simulink model "model_16_09_22"  (R2021a)
settings: Solver=FixedStepAuto  StartTime=0.0  StopTime=1370  FixedStep=0.01  RelTol=1e-3
values from neighbouring files (symbols this model uses):
  coord_0_ecef = [x_0_ecef, y_0_ecef, z_0_ecef]    [new_path_local_frame4_05_2022.m]
  dampPitchConst = 5    [Configuration_13_09_22FINESTRELLE.m]
  dampRollConst = 5    [Configuration_13_09_22FINESTRELLE.m]
  ECC = 0.0818191908426    [new_path_local_frame4_05_2022.m]
  FsGong = 8192    [matlabSounds.mat]
  FsHandel = 8192    [matlabSounds.mat]
  gainPitchTorque = -1000    [Configuration_13_09_22FINESTRELLE.m]
  gainRollTorque = -1000    [Configuration_13_09_22FINESTRELLE.m]
  indirect = 1    [Configuration_13_09_22FINESTRELLE.m]
  R_E = 6378137    [new_path_local_frame4_05_2022.m]
  RotationMatrix_NWU2ECEF = [-cos(lon0)*sin(lat0),  sin(lon0), cos(lon0)*cos(lat0) ... (first row only)    [new_path_local_frame4_05_2022.m]
  springPitchConst = 35    [Configuration_13_09_22FINESTRELLE.m]
  springRollConst = 35    [Configuration_13_09_22FINESTRELLE.m]
  timesPitch = 0.6    [Configuration_13_09_22FINESTRELLE.m]
  timesRoll = 0.6    [Configuration_13_09_22FINESTRELLE.m]
  yGong = [-0.00269844839217 -0.00449741398696 -0.00742073307848 -0.011018664268 -0.0128176298628 -0.0173150438498 -0.0222621992354 -0.0222621992354 -0.020013492242 -0.00921969867326 0.00449741398696 0.0101191814707 ... (42028 elements, 42028x1)]    [matlabSounds.mat]
  yHandel = [0 -0.00615680615681 -0.0750360750361 -0.0311688311688 0.00615680615681 0.0380952380952 0.0188552188552 -0.025012025012 -0.0311688311688 -0.0750360750361 -0.12582972583 -0.1443001443 ... (73113 elements, 73113x1)]    [matlabSounds.mat]
undefined symbols (not defined in the file or in its folder): DiscIntNeverNeededParam, f
libraries: cstblocks x7, simulink x6, instrumentlib x5
(part 2 of 2)

== matlab function model_16_09_22/Controllers/BuildMessage ==
  data: springRoll output; commandRollDiretto input; commandPitchDiretto input; frictionRoll output; dampRoll output; torqueRoll output; springPitch output; frictionPitch output; dampPitch output; torquePitch output; springYaw output; frictionYaw output; dampYaw output; torqueYaw output; springRollConst parameter; dampRollConst parameter; dampPitchConst parameter; springPitchConst parameter
function [springRoll, frictionRoll, dampRoll, torqueRoll,...
          springPitch, frictionPitch, dampPitch, torquePitch,...
          springYaw, frictionYaw, dampYaw, torqueYaw] = fcn(commandRollDiretto,commandPitchDiretto, springRollConst,...
                                                            dampRollConst,dampPitchConst, springPitchConst)
    
    springRoll = springRollConst;
    frictionRoll = 0; 
    dampRoll= dampRollConst; 
    torqueRoll = commandRollDiretto;
    
    springPitch = springPitchConst;
    frictionPitch = 0; 
    dampPitch = dampPitchConst; 
    torquePitch = commandPitchDiretto;
    
    springYaw = 0; 
    frictionYaw = 0; 
    dampYaw = 0; 
    torqueYaw = 0;

== matlab function model_16_09_22/ComputeError/ToWorkspace3/MATLAB Function ==
  data: intersectionPoint input; intersectionPointX output; intersectionPointY output; intersectionPointhZ output
function [intersectionPointX, intersectionPointY, intersectionPointhZ] = split(intersectionPoint)
          intersectionPointX = intersectionPoint(1);
          intersectionPointY = intersectionPoint(2);
          intersectionPointhZ = intersectionPoint(3);

== matlab function model_16_09_22/ComputeError/ToWorkspace2/MATLAB Function1 ==
  data: coordclock input; coordclockX output; coordclockY output; coordclockZ output
function [coordclockX, coordclockY, coordclockZ] = split(coordclock)
          coordclockX = coordclock(1);
          coordclockY = coordclock(2);
          coordclockZ = coordclock(3);

== matlab function model_16_09_22/ComputeError/ToWorkspace1/MATLAB Function2 ==
  data: posAircraft input; posAircraftX output; posAircraftY output; posAircraftZ output
function [posAircraftX, posAircraftY, posAircraftZ] = split(posAircraft)
          posAircraftX = posAircraft(1);
          posAircraftY = posAircraft(2);
          posAircraftZ = posAircraft(3);

== matlab function model_16_09_22/Controllers/MATLAB Function ==
  data: springRoll input; DataSend output; frictionRoll input; dampRoll input; torqueRoll input; springPitch input; frictionPitch input; dampPitch input; torquePitch input; springYaw input; frictionYaw input; dampYaw input; torqueYaw input
function DataSend  = fcn(springRoll, frictionRoll, dampRoll, torqueRoll, springPitch, frictionPitch, dampPitch, torquePitch, springYaw, frictionYaw, dampYaw, torqueYaw)

DataSend = [springRoll, frictionRoll, dampRoll, torqueRoll, springPitch, frictionPitch, dampPitch, torquePitch, springYaw, frictionYaw, dampYaw, torqueYaw];

== matlab function model_16_09_22/Controllers/Pitch1 ==
  data: h input; distPitch output
function distPitch = fcn(h)
    %PITCH   
    deadZoneZ = 0;  %[m]
    
    y = h ;
    
    if ((abs(h) > deadZoneZ) && (h > 0))
        errorheight = abs(abs(y) - deadZoneZ);
    elseif ((abs(h) > deadZoneZ) && (h < 0))
        errorheight = - abs(abs(y) - deadZoneZ); %y<0
    else
        errorheight = 0;
    end
    
    distPitch = errorheight;

== matlab function model_16_09_22/MagnitudeReceive/logStickDeflection/MATLAB Function1 ==
  data: stickDeflection input; stickDeflectionX output; stickDeflectionY output; stickDeflectionZ output
function [stickDeflectionX, stickDeflectionY, stickDeflectionZ] = split(stickDeflection)
          stickDeflectionX = stickDeflection(1);
          stickDeflectionY = stickDeflection(2);
          stickDeflectionZ = stickDeflection(3);

== matlab function model_16_09_22/MagnitudeReceive/logMotorTorque/MATLAB Function1 ==
  data: motorTorqueVector input; motorTorqueX output; motorTorqueY output
function [motorTorqueX, motorTorqueY] = split(motorTorqueVector)
          motorTorqueX = motorTorqueVector(1);
          motorTorqueY = motorTorqueVector(2);

== matlab function model_16_09_22/MATLAB Function ==
  data: yGong parameter; FsGong parameter; start input; yHandel parameter; FsHandel parameter
function audio(yGong, FsGong, start, yHandel, FsHandel)
         coder.extrinsic('sound');
         %DA METTERE NELLO SCRIPT load matlabSounds.mat
         if start == 1  
            sound(yGong, FsGong);
         elseif start == 2
           sound(yHandel, FsHandel);
         end
         
         
         %play(p, [1 (get(p, 'SampleRate') * 3)]);

== matlab function model_16_09_22/timeAnalysis/MATLAB Function1 ==
  data: WINDOWStimeSec output
   function WINDOWStimeSec = sysClock()
       coder.extrinsic('clock');

       H  =  0;
       MN = 0;
       S  =  0;
       dateTime = clock;
       H  = dateTime(4);
       MN = dateTime(5);
       S  = dateTime(6);
       
       % secondi dall'inizio dell'ora corrente
       WINDOWStimeSec = S + MN*60;
       
   end

== matlab function model_16_09_22/timeAnalysis/deBiaser ==
  data: u input; y output
function y = deBias(u)
persistent initVal

if isempty(initVal)
    initVal = u;
end


y = u - initVal;

== matlab function model_16_09_22/timeAnalysis/deBiaser1 ==
  data: u input; y output
function y = deBias(u)
persistent initVal

if isempty(initVal)
    initVal = u;
end


y = u - initVal;

== matlab function model_16_09_22/timeAnalysis/deBiaser2 ==
  data: u input; y output
function y = deBias(u)
persistent initVal

if isempty(initVal)
    initVal = u;
end


y = u - initVal;

== matlab function model_16_09_22/timeAnalysis/deBiaser3 ==
  data: u input; y output
function y = deBias(u)
persistent initVal

if isempty(initVal)
    initVal = u;
end


y = u - initVal;

== matlab function model_16_09_22/timeAnalysis/deBiaser4 ==
  data: u input; y output
function y = deBias(u)
persistent initVal

if isempty(initVal)
    initVal = u;
end


y = u - initVal;

== matlab function model_16_09_22/MATLAB Function1 ==
  data: start input; FsGong parameter; yGong parameter; yHandel parameter; FsHandel parameter
function audio(start, FsGong, yGong, yHandel, FsHandel)
         coder.extrinsic('sound');
         %DA METTERE NELLO SCRIPT load matlabSounds.mat
         if start == 1  
            sound(yGong, FsGong);
         elseif start == 1365
           sound(yHandel, FsHandel);
         end
end

== matlab function model_16_09_22/CoordinatesConversions/MATLAB Function ==
  data: lat input; coord_ecef output; lon input; alt input; ECC parameter; R_E parameter
function coord_ecef = geo2ecef(lat, lon, alt, ECC, R_E)
    %THIS BLOCK IS JUST TO UNDERSTAND IF AEROFLY ECEF SYSTEM IS ORIENTED IN
    %THE SAME WAY AS I WOULD DO IT


    %we already have lat lon in radians
    %coord_geo = [lat, lon, alt];

%     normal radius
    N = R_E / sqrt(1 - (ECC * sin(lat))^2);

%     coordinate transformation
    x_ecef = (N + alt) * cos(lat) * cos(lon);
    y_ecef = (N + alt) * cos(lat) * sin(lon);
    z_ecef = (N * (1 - ECC^2) + alt) * sin(lat);

    coord_ecef = [x_ecef, y_ecef, z_ecef];
end

== matlab function model_16_09_22/split message ==
  data: u input; flight_time output; lat output; lon output; height output; roll output; pitch output; yaw output; coord_ecef_aerofly output; altitude output; controls_roll_input output; controls_pitch_input output; controls_yaw_input output; aircraft_aileron output; aircraft_elevator output; aircraft_velocityX output; aircraft_velocityY output; aircraft_velocityZ output; UDPcounter output
function [flight_time, lat, lon, height, roll, pitch, yaw, ...
          coord_ecef_aerofly, altitude,controls_roll_input, controls_pitch_input, controls_yaw_input,...
          aircraft_aileron, aircraft_elevator, aircraft_velocityX, aircraft_velocityY, aircraft_velocityZ, UDPcounter] = split(u)
 
 
%// send binary data to matlab TO COUNT IN MATLAB ADD 1
% 	gAircraftData2MatlabBuffer[0] = lfFlightTimeS;
% 
% 	gAircraftData2MatlabBuffer[1] = aircraft_position.x;
% 	gAircraftData2MatlabBuffer[2] = aircraft_position.y;
% 	gAircraftData2MatlabBuffer[3] = aircraft_position.z;
% 
% 	gAircraftData2MatlabBuffer[4] = aircraft_latitude;
% 	gAircraftData2MatlabBuffer[5] = aircraft_longitude;
% 
% 	gAircraftData2MatlabBuffer[6] = aircraft_height;
% 
% 	gAircraftData2MatlabBuffer[7] = aircraft_altitude;
% 
% 	gAircraftData2MatlabBuffer[8] = aircraft_bank;
% 	gAircraftData2MatlabBuffer[9] = aircraft_pitch;
% 	gAircraftData2MatlabBuffer[10] = aircraft_heading;
% 	gAircraftData2MatlabBuffer[11] = controls_roll_input;
% 	gAircraftData2MatlabBuffer[12] = controls_pitch_input;
% 	gAircraftData2MatlabBuffer[13] = controls_yaw_input;
% 	//gAircraftData2MatlabBuffer[14] = controls_roll_input_offset;
% 	//gAircraftData2MatlabBuffer[15] = controls_pitch_input_offset;
% 	gAircraftData2MatlabBuffer[14] = aircraft_aileron;
% 	gAircraftData2MatlabBuffer[15] = aircraft_elevator;
% 	gAircraftData2MatlabBuffer[16] = aircraft_velocity.x;
% 	gAircraftData2MatlabBuffer[17] = aircraft_velocity.y;
% 	gAircraftData2MatlabBuffer[18] = aircraft_velocity.z;
% 	
% 
% 	// ...
% 	gAircraftData2MatlabBuffer[19] = nUdpCounter;


    flight_time = u(1);
    x_pos = u(2);
    y_pos = u(3);
    z_pos = - u(4);
    coord_ecef_aerofly = [x_pos, y_pos, - z_pos];
    
    lat = u(5);
    lon = u(6);
    height = u(7);
    
    altitude = u(8);
    
    roll = rad2deg(u(9));
    pitch = - rad2deg(u(10));
    %pay attention the conversion is made just here and not in the logfile
    %this way the angle will be referred to the north and counted clockwise
    %for now we don't use it, but pay attention to the local frame and the
    %reference systems of the other angles if using them together for the
    %feedback
    yaw = 360 - rad2deg(u(11)) + 90;
    
    controls_roll_input = u(12);
    controls_pitch_input = u(13);
    controls_yaw_input = u(14);
        
    aircraft_aileron = u(15);
    aircraft_elevator = u(16);
    
    aircraft_velocityX = u(17);
    aircraft_velocityY = u(18);
    aircraft_velocityZ = u(19);
    
    UDPcounter = u(20);
    
    
end

== matlab function model_16_09_22/ComputeError/ToWorkspace4/MATLAB Function1 ==
  data: aircraft2path input; aircraft2pathX output; aircraft2pathY output; aircraft2pathZ output
function [aircraft2pathX, aircraft2pathY, aircraft2pathZ] = split(aircraft2path)
          aircraft2pathX = aircraft2path(1);
          aircraft2pathY = aircraft2path(2);
          aircraft2pathZ = aircraft2path(3);

== matlab function model_16_09_22/ComputeError/ComputeValidIndex ==
  data: startIndex output; stopIndex output; min_valid_index output; min_valid_theta output; min_valid_coord_path output; min_valid_tangent output; eps_Deg output; min_valid_aircraft2path output; norm_min_valid_aircraft2path output; g_Coordinates data_store_memory; plane_coord_nwu input; R parameter

function [startIndex, stopIndex, min_valid_index, ...
          min_valid_theta, min_valid_coord_path, min_valid_tangent, eps_Deg, ...
          min_valid_aircraft2path, norm_min_valid_aircraft2path] = fcn(plane_coord_nwu, R)

global g_Coordinates
persistent p_epsDeg; if isempty(p_epsDeg) p_epsDeg = 120.0; end
persistent p_prev_min_index ; if isempty(p_prev_min_index) p_prev_min_index = 1; end
persistent p_act_min_index ; if isempty(p_act_min_index) p_act_min_index = 1; end
persistent p_start; if isempty(p_start) p_start = true; end
persistent p_tangent_min; if isempty(p_tangent_min) p_tangent_min = [0, 0, 0]; end
persistent p_coord_path_min; if isempty(p_coord_path_min) p_coord_path_min = [0, 0, 0]; end
persistent p_min_valid_aircraft2path; if isempty(p_min_valid_aircraft2path) p_min_valid_aircraft2path = [0, 0, 0]; end

nSteps = g_Coordinates.Steps;

%init some variables
n90DegCounter = 0; 
ThetaDeg_out = 10000000;
min_valid_theta = ThetaDeg_out;
comparing_norm_aircraft2path = 99999999;

sinew = 2*R*sin(pi/nSteps);
section_width = 30;
scaler = 10000.0;
limiter = scaler * R / (180.0 * nSteps);

%taking actual position in local frame
pos_airplane = plane_coord_nwu;

if p_start == true
    startIndex = 1;
    stopIndex = nSteps;
else
    % take last found index and set a "section-window" around it to reduce
    % the found results an get the "right" solution
    startIndex = p_prev_min_index - section_width/2;
    if startIndex < 0
       startIndex = startIndex + nSteps;
    end
    if startIndex == 0
        startIndex = 1;
    end
    
    stopIndex = p_prev_min_index + section_width/2;
    if stopIndex > nSteps
        stopIndex = stopIndex - nSteps;
    end
end

%i is the index for iterating through the already generated path(g_Coordinates.Trajectory)
i = startIndex;

 while (true)
    %taking coordinates from global variable
    %path is defined in local frame nwu
    x_clock = g_Coordinates.Trajectory(i).x;
    y_clock = g_Coordinates.Trajectory(i).y;
    z_clock = g_Coordinates.Trajectory(i).z;
    coord_clock_on_path = [x_clock, y_clock, z_clock];
    %derivatives, tangents to each point of the path
    dx_clock = g_Coordinates.Trajectory(i).dx;
    dy_clock = g_Coordinates.Trajectory(i).dy;
    dz_clock = g_Coordinates.Trajectory(i).dz;
    d_clock = [dx_clock, dy_clock, dz_clock]; %ATTENZIONE FORSE DEVI FARE LA NORMA
    
    %distance vector between plane and path
    %the sign isn´t importante, we use this vector to compute
    %the scalar product and get it when it's almost zero
    %according to the coordinate system, h has to be always positive from plane to path
    aircraft2path = - (pos_airplane - coord_clock_on_path);
    normAircraft2Path = norm(aircraft2path);
    normXYAircraft2Path = sqrt( aircraft2path(1)^2 + aircraft2path(2)^2 );
         
    %computing scalar product between the tangent to the circle
    %and the distance vector from the airplane to the circle
    C = dot(d_clock, aircraft2path); % scalarproduct is zero when vectors are 90 degrees
    
    %computing angle between the two vectors
    CosTheta = C/((norm(d_clock))* normAircraft2Path);
    Theta_deg = real(acosd(CosTheta));
    
    %find the angle 90 deg between plane-vector and path-vector if
    %aircraft is not on the path yet
    %when aircraft2path is a small vector we accept every angle, the program
    %should just look for the smallest distance of the aircraft to the path
    if  (( (abs(90 - Theta_deg)<= p_epsDeg) || (normXYAircraft2Path < sinew/2)))

        ThetaDeg_out = Theta_deg;
        %counter used for debugging, we need it to check how many
        %times theta is around 90
        n90DegCounter = n90DegCounter + 1; %it counts every time it does the loop
        g_Coordinates.n90DegCounter = n90DegCounter;
        
        %compute aircraft2path for each pathClock when theta is 90° or
        %normXYAircraft2Path < sinew/2, we will call this case "valid"
        norm_valid_aircraft2path = norm(aircraft2path);
        
        %find minimum value of the distance between aircraft and path,
        %in the "valid" case defined above
        if  norm_valid_aircraft2path < comparing_norm_aircraft2path
            comparing_norm_aircraft2path = norm_valid_aircraft2path;
            p_act_min_index = i;
            min_valid_theta = ThetaDeg_out;
            p_tangent_min = d_clock; %tangent has to be normalized in the next block
            p_coord_path_min = coord_clock_on_path;
            p_min_valid_aircraft2path = aircraft2path;         
        end
    end
    
    %detect end of loop 
    if (i == stopIndex)
       break;
    end
    
    % set next iteration
    i = i + 1;
    
    % manage transition at max steps
    if (i == nSteps+1)
        i = 1;
    end
    
 end % end while

% set values for the next simulink cycle
p_start = false;
p_prev_min_index = p_act_min_index;

%window changes depending on how far we are away from the path
if (comparing_norm_aircraft2path > (sinew/2) && n90DegCounter > 0)
    p_epsDeg = scaler*R/((comparing_norm_aircraft2path + limiter)*nSteps); %version Harald
end

% set output variables
min_valid_index = p_act_min_index;
eps_Deg = p_epsDeg;
min_valid_coord_path = p_coord_path_min;
min_valid_tangent = p_tangent_min;
min_valid_aircraft2path = p_min_valid_aircraft2path;
norm_min_valid_aircraft2path = norm(min_valid_aircraft2path);
end % function

% end of file
